simulink model "gm_uz_count_switching"  (R2024a)
settings: Solver=FixedStepDiscrete  StartTime=0.0  StopTime=350e-6  RelTol=1e-3
libraries: hdlsllib x9, simulink x1
settings Model: Creator=josef  LastModifiedBy=josef
settings SolverCC: AlgebraicLoopSolver=TrustRegion
settings DataIOCC: LimitDataPoints=on  SaveOutput=off  SaveTime=off
settings OptimizationCC: BlockReduction=off  ConditionallyExecuteInputs=off  DefaultParameterBehavior=Inlined  InheritOutputTypeSmallerThanSingle=on  LifeSpan=inf
settings DebuggingCC: AlgebraicLoopMsg=error  InheritedTsInSrcMsg=none  SingleTaskRateTransMsg=error  UnconnectedInputMsg=warning  UnconnectedOutputMsg=warning  UnconnectedLineMsg=warning  AllowSymbolicDim=off  StrictBusMsg=ErrorOnBusTreatedAsVector  SFUnexpectedBacktrackingDiag=warning  SFNoUnconditionalDefaultTransitionDiag=warning  SFExecutionAtInitializationDiag=none  ArithmeticOperatorsInVariantConditions=warning
settings HardwareCC: ProdBitPerPointer=32  ProdBitPerSizeT=32  ProdBitPerPtrDiffT=32  ProdLargestAtomicFloat=None  ProdIntDivRoundTo=Undefined  ProdEndianess=Unspecified  ProdWordSize=32  ProdHWDeviceType=ASIC/FPGA->ASIC/FPGA  ProdEqTarget=off
settings ModelReferenceCC: EnableRefExpFcnMdlSchedulingChecks=on
settings SFSimCC: SimUseLocalCustomCode=off  CustomCodeUndefinedFunction=UseInterfaceOnly
settings RTWCC: RTWUseLocalCustomCode=off  GPUComputeCapability=3.5
settings CodeAppCC: StateflowObjectComments=on
settings GRTTargetCC: TargetLangStandard=C89/C90 (ANSI)
settings ConfigComp: CovScope=ReferencedModels  CovMetricSettings=dw  CovSaveCumulativeToWorkspaceVar=on  CovSaveSingleToWorkspaceVar=on  CovExternalEMLEnable=off  CovSFcnEnable=off

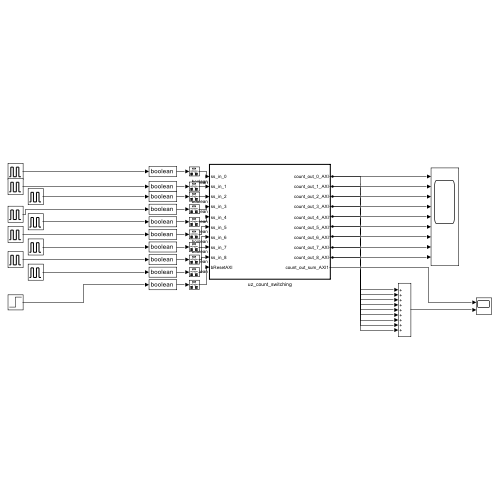
[thumbnail: Simulink's stored preview of the top-level diagram]
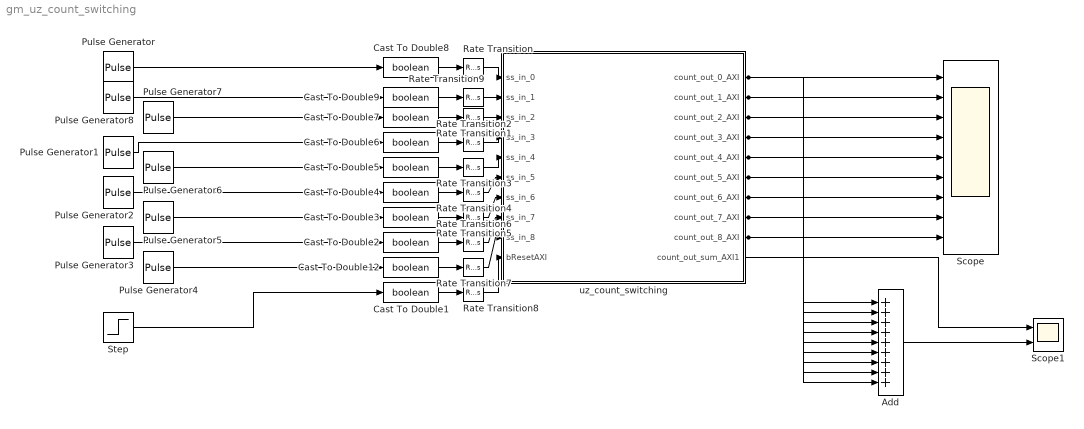
== system gm_uz_count_switching ==
  Add : Sum  Inputs=+++++++++
  Cast To Double{1..9,12} (10 alike) : DataTypeConversion  OutDataTypeStr=boolean  SaturateOnIntegerOverflow=off  RndMeth=Floor
  Pulse Generator{,1..5,7..8} (8 alike) : DiscretePulseGenerator  PulseType=Time based  Period=100e-6  PulseWidth=5
  Pulse Generator6 : DiscretePulseGenerator  PulseType=Time based  Period=50e-6  PulseWidth=5
  Rate Transition{,1..9} (10 alike) : RateTransition  OutPortSampleTime=1/100000000
  Scope : Scope  NumInputPorts=9
  Scope1 : Scope  NumInputPorts=2
  Step : Step  Time=2e-4  SampleTime=0
  uz_count_switching : Subsystem  TreatAsAtomicUnit=on
  wires:
  Pulse Generator8/1 -> Cast To Double9/1
  Cast To Double9/1 -> Rate Transition9/1
  Rate Transition9/1 -> uz_count_switching/2(ss_in_1)
  Rate Transition8/1 -> uz_count_switching/10(bResetAXI)
  Rate Transition7/1 -> uz_count_switching/9(ss_in_8)
  Rate Transition6/1 -> uz_count_switching/8(ss_in_7)
  Rate Transition5/1 -> uz_count_switching/7(ss_in_6)
  Rate Transition4/1 -> uz_count_switching/6(ss_in_5)
  Rate Transition3/1 -> uz_count_switching/5(ss_in_4)
  Rate Transition2/1 -> uz_count_switching/4(ss_in_3)
  Rate Transition1/1 -> uz_count_switching/3(ss_in_2)
  Cast To Double8/1 -> Rate Transition/1
  Cast To Double7/1 -> Rate Transition1/1
  Cast To Double6/1 -> Rate Transition2/1
  Cast To Double5/1 -> Rate Transition3/1
  Cast To Double4/1 -> Rate Transition4/1
  Cast To Double3/1 -> Rate Transition5/1
  Cast To Double2/1 -> Rate Transition6/1
  Cast To Double1/1 -> Rate Transition8/1
  Cast To Double12/1 -> Rate Transition7/1
  Rate Transition/1 -> uz_count_switching/1(ss_in_0)
  Pulse Generator5/1 -> Cast To Double3/1
  Pulse Generator6/1 -> Cast To Double5/1
  Pulse Generator7/1 -> Cast To Double7/1
  Pulse Generator4/1 -> Cast To Double12/1
  Pulse Generator3/1 -> Cast To Double2/1
  Pulse Generator2/1 -> Cast To Double4/1
  Pulse Generator1/1 -> Cast To Double6/1
  Pulse Generator/1 -> Cast To Double8/1
  Step/1 -> Cast To Double1/1
  Add/1 -> Scope1/2
  uz_count_switching/10(count_out_sum_AXI1) -> Scope1/1
  uz_count_switching/9(count_out_8_AXI) -> Scope/9, Add/9
  uz_count_switching/8(count_out_7_AXI) -> Scope/8, Add/8
  uz_count_switching/7(count_out_6_AXI) -> Scope/7, Add/7
  uz_count_switching/6(count_out_5_AXI) -> Scope/6, Add/6
  uz_count_switching/5(count_out_4_AXI) -> Scope/5, Add/5
  uz_count_switching/4(count_out_3_AXI) -> Scope/4, Add/4
  uz_count_switching/3(count_out_2_AXI) -> Scope/3, Add/3
  uz_count_switching/2(count_out_1_AXI) -> Scope/2, Add/2
  uz_count_switching/1(count_out_0_AXI) -> Scope/1, Add/1

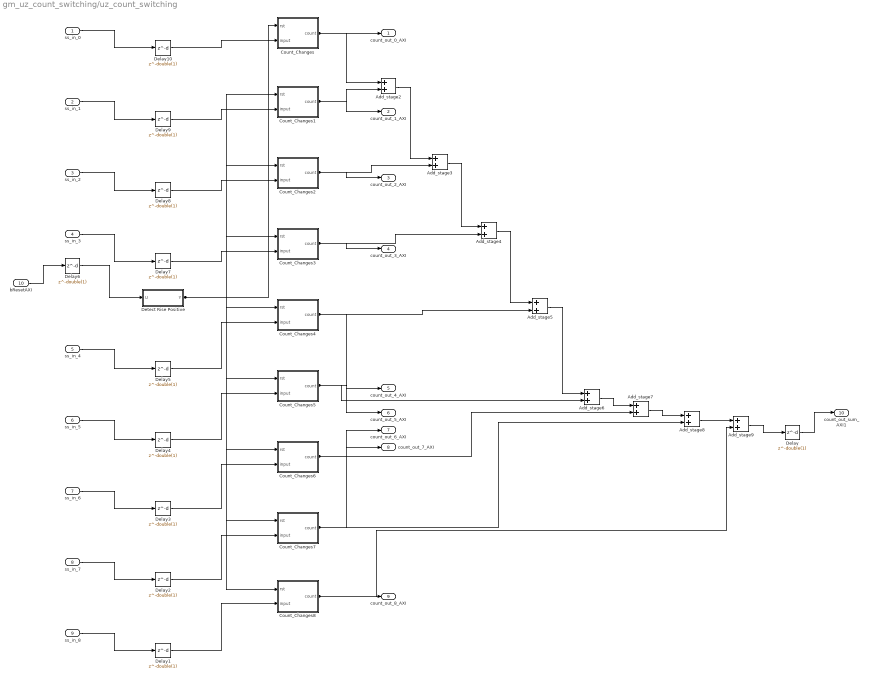
== system gm_uz_count_switching/uz_count_switching ==
  ss_in_0 : Inport  OutDataTypeStr=boolean  PortDimensions=1  SampleTime=1e-08
  ss_in_1 : Inport  Port=2  OutDataTypeStr=boolean  PortDimensions=1  SampleTime=1e-08
  ss_in_2 : Inport  Port=3  OutDataTypeStr=boolean  PortDimensions=1  SampleTime=1e-08
  ss_in_3 : Inport  Port=4  OutDataTypeStr=boolean  PortDimensions=1  SampleTime=1e-08
  ss_in_4 : Inport  Port=5  OutDataTypeStr=boolean  PortDimensions=1  SampleTime=1e-08
  ss_in_5 : Inport  Port=6  OutDataTypeStr=boolean  PortDimensions=1  SampleTime=1e-08
  ss_in_6 : Inport  Port=7  OutDataTypeStr=boolean  PortDimensions=1  SampleTime=1e-08
  ss_in_7 : Inport  Port=8  OutDataTypeStr=boolean  PortDimensions=1  SampleTime=1e-08
  ss_in_8 : Inport  Port=9  OutDataTypeStr=boolean  PortDimensions=1  SampleTime=1e-08
  bResetAXI : Inport  Port=10  OutDataTypeStr=boolean  PortDimensions=1  SampleTime=1e-08
  Add_stage2 : Sum  OutDataTypeStr=fixdt(0, 33, 0)  AccumDataTypeStr=uint32  SampleTime=1e-08
  Add_stage3 : Sum  OutDataTypeStr=fixdt(0, 34, 0)  AccumDataTypeStr=uint32  SampleTime=1e-08
  Add_stage4 : Sum  OutDataTypeStr=fixdt(0, 35, 0)  AccumDataTypeStr=uint32  SampleTime=1e-08
  Add_stage5 : Sum  OutDataTypeStr=fixdt(0, 36, 0)  AccumDataTypeStr=uint32  SampleTime=1e-08
  Add_stage6 : Sum  OutDataTypeStr=fixdt(0, 37, 0)  AccumDataTypeStr=uint32  SampleTime=1e-08
  Add_stage7 : Sum  OutDataTypeStr=fixdt(0, 38, 0)  AccumDataTypeStr=uint32  SampleTime=1e-08
  Add_stage8 : Sum  OutDataTypeStr=fixdt(0, 39, 0)  AccumDataTypeStr=uint32  SampleTime=1e-08
  Add_stage9 : Sum  OutDataTypeStr=uint32  AccumDataTypeStr=uint32  SampleTime=1e-08
  Count_Changes : Subsystem
  Count_Changes1 : Subsystem
  Count_Changes2 : Subsystem
  Count_Changes3 : Subsystem
  Count_Changes4 : Subsystem
  Count_Changes5 : Subsystem
  Count_Changes6 : Subsystem
  Count_Changes7 : Subsystem
  Count_Changes8 : Subsystem
  Delay{,1..10} (11 alike) : Delay  DelayLength=double(1)  InitialCondition=0  SampleTime=1e-08
  Detect Rise Positive : Subsystem  mask(Detect Rise Positive){vinit=double(0), InputProcessing=Elements as channels (sample based), OutDataTypeStr=boolean}
      mask prompts: vinit "Simulink:masks:InitialCondition_MP"; InputProcessing "Simulink:masks:InputProcessing_MP"; OutDataTypeStr "Simulink:masks:OutputDataType_MP"
      mask help: Simulink:masks:DetectRisePositive_MD
      mask init:
      | InputProcessing = 'Elements as channels (sample based)';
      | OutDataTypeStr = 'boolean';
      | vinit = double(0);
      mask TypeOptions InputProcessing: Simulink:masks:ColumnsAsChannelsFrameBased | Simulink:masks:ElementsAsChannelsSampleBased
      mask TypeOptions OutDataTypeStr: Simulink:masks:uint8 | Simulink:masks:boolean
      mask Display: fprintf('U > 0\n&  NOT\nU/z > 0')
  count_out_0_AXI : Outport  SampleTime=1e-08  VectorParamsAs1DForOutWhenUnconnected=off
  count_out_1_AXI : Outport  Port=2  SampleTime=1e-08  VectorParamsAs1DForOutWhenUnconnected=off
  count_out_2_AXI : Outport  Port=3  SampleTime=1e-08  VectorParamsAs1DForOutWhenUnconnected=off
  count_out_3_AXI : Outport  Port=4  SampleTime=1e-08  VectorParamsAs1DForOutWhenUnconnected=off
  count_out_4_AXI : Outport  Port=5  SampleTime=1e-08  VectorParamsAs1DForOutWhenUnconnected=off
  count_out_5_AXI : Outport  Port=6  SampleTime=1e-08  VectorParamsAs1DForOutWhenUnconnected=off
  count_out_6_AXI : Outport  Port=7  SampleTime=1e-08  VectorParamsAs1DForOutWhenUnconnected=off
  count_out_7_AXI : Outport  Port=8  SampleTime=1e-08  VectorParamsAs1DForOutWhenUnconnected=off
  count_out_8_AXI : Outport  Port=9  SampleTime=1e-08  VectorParamsAs1DForOutWhenUnconnected=off
  count_out_sum_AXI1 : Outport  Port=10  SampleTime=1e-08  VectorParamsAs1DForOutWhenUnconnected=off
  wires:
  ss_in_0/1 -> Delay10/1
  ss_in_1/1 -> Delay9/1
  ss_in_2/1 -> Delay8/1
  ss_in_3/1 -> Delay7/1
  ss_in_4/1 -> Delay5/1
  ss_in_5/1 -> Delay4/1
  ss_in_6/1 -> Delay3/1
  ss_in_7/1 -> Delay2/1
  ss_in_8/1 -> Delay1/1
  bResetAXI/1 -> Delay6/1
  Add_stage9/1 -> Delay/1
  Count_Changes/1(count) -> Add_stage2/1, count_out_0_AXI/1
  Count_Changes1/1(count) -> Add_stage2/2, count_out_1_AXI/1
  Count_Changes2/1(count) -> Add_stage3/2, count_out_2_AXI/1
  Count_Changes3/1(count) -> Add_stage4/2, count_out_3_AXI/1
  Count_Changes4/1(count) -> Add_stage5/2, count_out_4_AXI/1
  Count_Changes5/1(count) -> Add_stage6/2, count_out_5_AXI/1
  Count_Changes6/1(count) -> Add_stage7/2, count_out_6_AXI/1
  Count_Changes7/1(count) -> Add_stage8/2, count_out_7_AXI/1
  Count_Changes8/1(count) -> Add_stage9/2, count_out_8_AXI/1
  Delay/1 -> count_out_sum_AXI1/1
  Delay1/1 -> Count_Changes8/2(input)
  Delay10/1 -> Count_Changes/2(input)
  Delay2/1 -> Count_Changes7/2(input)
  Delay3/1 -> Count_Changes6/2(input)
  Delay4/1 -> Count_Changes5/2(input)
  Delay5/1 -> Count_Changes4/2(input)
  Delay6/1 -> Detect Rise Positive/1(U)
  Delay7/1 -> Count_Changes3/2(input)
  Delay8/1 -> Count_Changes2/2(input)
  Delay9/1 -> Count_Changes1/2(input)
  Detect Rise Positive/1(Y) -> Count_Changes/1(rst), Count_Changes1/1(rst), Count_Changes2/1(rst), Count_Changes3/1(rst), Count_Changes4/1(rst), Count_Changes5/1(rst), Count_Changes6/1(rst), Count_Changes7/1(rst), Count_Changes8/1(rst)
  Add_stage2/1 -> Add_stage3/1
  Add_stage3/1 -> Add_stage4/1
  Add_stage4/1 -> Add_stage5/1
  Add_stage5/1 -> Add_stage6/1
  Add_stage6/1 -> Add_stage7/1
  Add_stage7/1 -> Add_stage8/1
  Add_stage8/1 -> Add_stage9/1

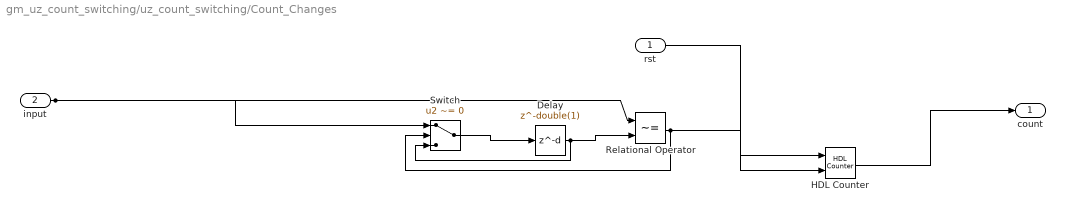
== system gm_uz_count_switching/uz_count_switching/Count_Changes ==
  rst : Inport  OutDataTypeStr=boolean  PortDimensions=1  SampleTime=1e-08
  input : Inport  Port=2  OutDataTypeStr=boolean  PortDimensions=1  SampleTime=1e-08
  Delay : Delay  DelayLength=double(1)  InitialCondition=0  SampleTime=1e-08
  HDL Counter : hdlsllib/Sources/HDL Counter  CountType=Free running  CountInit=0  CountStep=1  CountMax=25  CountFromType=Initial value  CountFrom=0  CountResetPort=on  CountLoadPort=off  CountEnbPort=on  CountDirPort=off  CountHitOutputPort=off  CountDataType=Unsigned  CountWordLen=CounterWordLength  CountFracLen=0  CountSampTime=1
  Relational Operator : RelationalOperator  Operator=~=  OutDataTypeStr=boolean  SampleTime=1e-08  InputSameDT=off
  Switch : Switch  Criteria=u2 ~= 0  Threshold=double(0)  OutDataTypeStr=boolean  SampleTime=1e-08  SaturateOnIntegerOverflow=off  InputSameDT=off
  count : Outport  SampleTime=1e-08
  wires:
  rst/1 -> HDL Counter/1
  input/1 -> Switch/1, Relational Operator/1
  Delay/1 -> Switch/3, Relational Operator/2
  HDL Counter/1 -> count/1
  Relational Operator/1 -> Switch/2, HDL Counter/2
  Switch/1 -> Delay/1

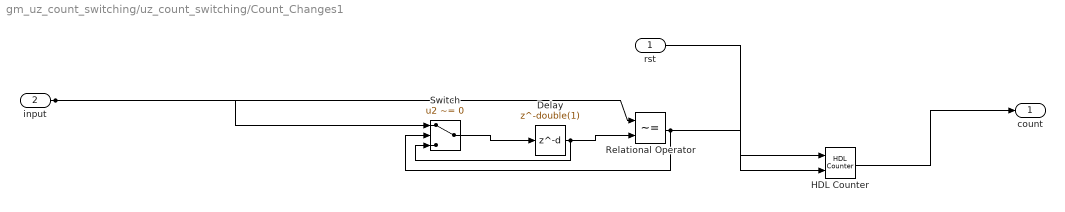
== system gm_uz_count_switching/uz_count_switching/Count_Changes1 ==
  rst : Inport  OutDataTypeStr=boolean  PortDimensions=1  SampleTime=1e-08
  input : Inport  Port=2  OutDataTypeStr=boolean  PortDimensions=1  SampleTime=1e-08
  Delay : Delay  DelayLength=double(1)  InitialCondition=0  SampleTime=1e-08
  HDL Counter : hdlsllib/Sources/HDL Counter  CountType=Free running  CountInit=0  CountStep=1  CountMax=25  CountFromType=Initial value  CountFrom=0  CountResetPort=on  CountLoadPort=off  CountEnbPort=on  CountDirPort=off  CountHitOutputPort=off  CountDataType=Unsigned  CountWordLen=CounterWordLength  CountFracLen=0  CountSampTime=1
  Relational Operator : RelationalOperator  Operator=~=  OutDataTypeStr=boolean  SampleTime=1e-08  InputSameDT=off
  Switch : Switch  Criteria=u2 ~= 0  Threshold=double(0)  OutDataTypeStr=boolean  SampleTime=1e-08  SaturateOnIntegerOverflow=off  InputSameDT=off
  count : Outport  SampleTime=1e-08
  wires:
  rst/1 -> HDL Counter/1
  input/1 -> Switch/1, Relational Operator/1
  Delay/1 -> Switch/3, Relational Operator/2
  HDL Counter/1 -> count/1
  Relational Operator/1 -> Switch/2, HDL Counter/2
  Switch/1 -> Delay/1

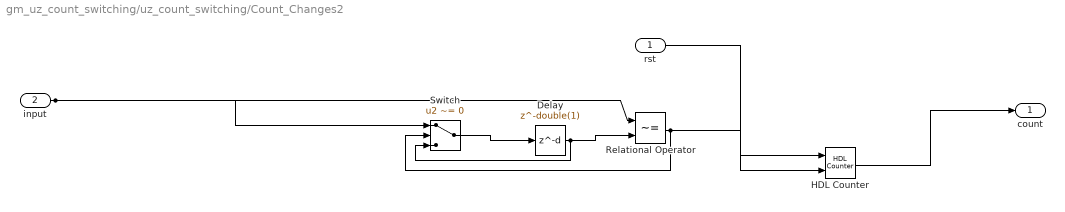
== system gm_uz_count_switching/uz_count_switching/Count_Changes2 ==
  rst : Inport  OutDataTypeStr=boolean  PortDimensions=1  SampleTime=1e-08
  input : Inport  Port=2  OutDataTypeStr=boolean  PortDimensions=1  SampleTime=1e-08
  Delay : Delay  DelayLength=double(1)  InitialCondition=0  SampleTime=1e-08
  HDL Counter : hdlsllib/Sources/HDL Counter  CountType=Free running  CountInit=0  CountStep=1  CountMax=25  CountFromType=Initial value  CountFrom=0  CountResetPort=on  CountLoadPort=off  CountEnbPort=on  CountDirPort=off  CountHitOutputPort=off  CountDataType=Unsigned  CountWordLen=CounterWordLength  CountFracLen=0  CountSampTime=1
  Relational Operator : RelationalOperator  Operator=~=  OutDataTypeStr=boolean  SampleTime=1e-08  InputSameDT=off
  Switch : Switch  Criteria=u2 ~= 0  Threshold=double(0)  OutDataTypeStr=boolean  SampleTime=1e-08  SaturateOnIntegerOverflow=off  InputSameDT=off
  count : Outport  SampleTime=1e-08
  wires:
  rst/1 -> HDL Counter/1
  input/1 -> Switch/1, Relational Operator/1
  Delay/1 -> Switch/3, Relational Operator/2
  HDL Counter/1 -> count/1
  Relational Operator/1 -> Switch/2, HDL Counter/2
  Switch/1 -> Delay/1

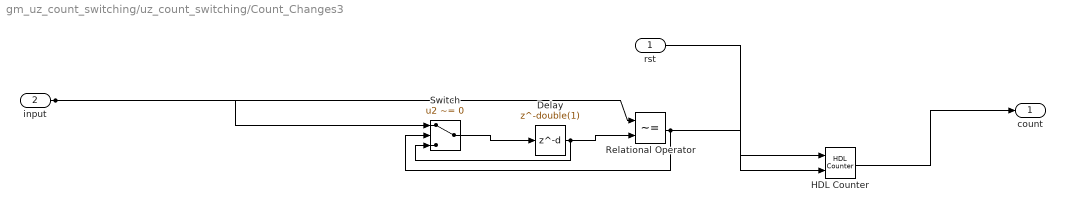
== system gm_uz_count_switching/uz_count_switching/Count_Changes3 ==
  rst : Inport  OutDataTypeStr=boolean  PortDimensions=1  SampleTime=1e-08
  input : Inport  Port=2  OutDataTypeStr=boolean  PortDimensions=1  SampleTime=1e-08
  Delay : Delay  DelayLength=double(1)  InitialCondition=0  SampleTime=1e-08
  HDL Counter : hdlsllib/Sources/HDL Counter  CountType=Free running  CountInit=0  CountStep=1  CountMax=25  CountFromType=Initial value  CountFrom=0  CountResetPort=on  CountLoadPort=off  CountEnbPort=on  CountDirPort=off  CountHitOutputPort=off  CountDataType=Unsigned  CountWordLen=CounterWordLength  CountFracLen=0  CountSampTime=1
  Relational Operator : RelationalOperator  Operator=~=  OutDataTypeStr=boolean  SampleTime=1e-08  InputSameDT=off
  Switch : Switch  Criteria=u2 ~= 0  Threshold=double(0)  OutDataTypeStr=boolean  SampleTime=1e-08  SaturateOnIntegerOverflow=off  InputSameDT=off
  count : Outport  SampleTime=1e-08
  wires:
  rst/1 -> HDL Counter/1
  input/1 -> Switch/1, Relational Operator/1
  Delay/1 -> Switch/3, Relational Operator/2
  HDL Counter/1 -> count/1
  Relational Operator/1 -> Switch/2, HDL Counter/2
  Switch/1 -> Delay/1

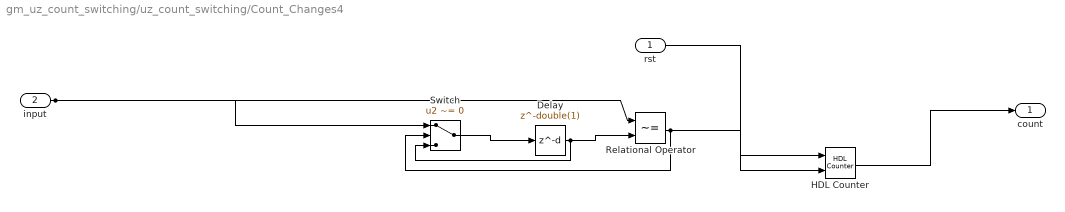
== system gm_uz_count_switching/uz_count_switching/Count_Changes4 ==
  rst : Inport  OutDataTypeStr=boolean  PortDimensions=1  SampleTime=1e-08
  input : Inport  Port=2  OutDataTypeStr=boolean  PortDimensions=1  SampleTime=1e-08
  Delay : Delay  DelayLength=double(1)  InitialCondition=0  SampleTime=1e-08
  HDL Counter : hdlsllib/Sources/HDL Counter  CountType=Free running  CountInit=0  CountStep=1  CountMax=25  CountFromType=Initial value  CountFrom=0  CountResetPort=on  CountLoadPort=off  CountEnbPort=on  CountDirPort=off  CountHitOutputPort=off  CountDataType=Unsigned  CountWordLen=CounterWordLength  CountFracLen=0  CountSampTime=1
  Relational Operator : RelationalOperator  Operator=~=  OutDataTypeStr=boolean  SampleTime=1e-08  InputSameDT=off
  Switch : Switch  Criteria=u2 ~= 0  Threshold=double(0)  OutDataTypeStr=boolean  SampleTime=1e-08  SaturateOnIntegerOverflow=off  InputSameDT=off
  count : Outport  SampleTime=1e-08
  wires:
  rst/1 -> HDL Counter/1
  input/1 -> Switch/1, Relational Operator/1
  Delay/1 -> Switch/3, Relational Operator/2
  HDL Counter/1 -> count/1
  Relational Operator/1 -> Switch/2, HDL Counter/2
  Switch/1 -> Delay/1

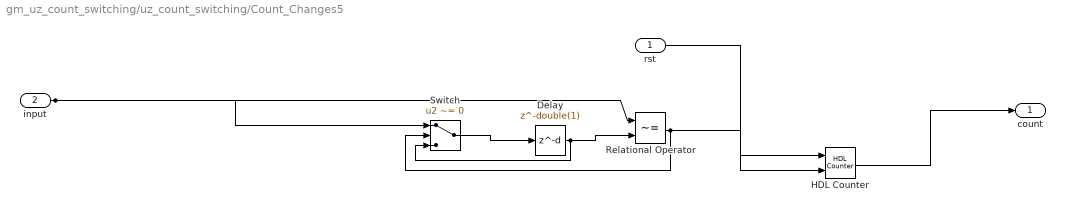
== system gm_uz_count_switching/uz_count_switching/Count_Changes5 ==
  rst : Inport  OutDataTypeStr=boolean  PortDimensions=1  SampleTime=1e-08
  input : Inport  Port=2  OutDataTypeStr=boolean  PortDimensions=1  SampleTime=1e-08
  Delay : Delay  DelayLength=double(1)  InitialCondition=0  SampleTime=1e-08
  HDL Counter : hdlsllib/Sources/HDL Counter  CountType=Free running  CountInit=0  CountStep=1  CountMax=25  CountFromType=Initial value  CountFrom=0  CountResetPort=on  CountLoadPort=off  CountEnbPort=on  CountDirPort=off  CountHitOutputPort=off  CountDataType=Unsigned  CountWordLen=CounterWordLength  CountFracLen=0  CountSampTime=1
  Relational Operator : RelationalOperator  Operator=~=  OutDataTypeStr=boolean  SampleTime=1e-08  InputSameDT=off
  Switch : Switch  Criteria=u2 ~= 0  Threshold=double(0)  OutDataTypeStr=boolean  SampleTime=1e-08  SaturateOnIntegerOverflow=off  InputSameDT=off
  count : Outport  SampleTime=1e-08
  wires:
  rst/1 -> HDL Counter/1
  input/1 -> Switch/1, Relational Operator/1
  Delay/1 -> Switch/3, Relational Operator/2
  HDL Counter/1 -> count/1
  Relational Operator/1 -> Switch/2, HDL Counter/2
  Switch/1 -> Delay/1

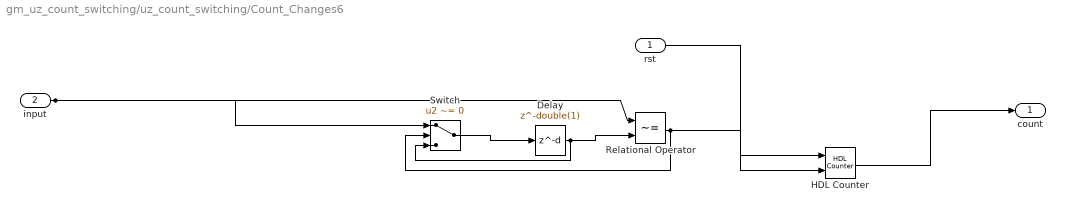
== system gm_uz_count_switching/uz_count_switching/Count_Changes6 ==
  rst : Inport  OutDataTypeStr=boolean  PortDimensions=1  SampleTime=1e-08
  input : Inport  Port=2  OutDataTypeStr=boolean  PortDimensions=1  SampleTime=1e-08
  Delay : Delay  DelayLength=double(1)  InitialCondition=0  SampleTime=1e-08
  HDL Counter : hdlsllib/Sources/HDL Counter  CountType=Free running  CountInit=0  CountStep=1  CountMax=25  CountFromType=Initial value  CountFrom=0  CountResetPort=on  CountLoadPort=off  CountEnbPort=on  CountDirPort=off  CountHitOutputPort=off  CountDataType=Unsigned  CountWordLen=CounterWordLength  CountFracLen=0  CountSampTime=1
  Relational Operator : RelationalOperator  Operator=~=  OutDataTypeStr=boolean  SampleTime=1e-08  InputSameDT=off
  Switch : Switch  Criteria=u2 ~= 0  Threshold=double(0)  OutDataTypeStr=boolean  SampleTime=1e-08  SaturateOnIntegerOverflow=off  InputSameDT=off
  count : Outport  SampleTime=1e-08
  wires:
  rst/1 -> HDL Counter/1
  input/1 -> Switch/1, Relational Operator/1
  Delay/1 -> Switch/3, Relational Operator/2
  HDL Counter/1 -> count/1
  Relational Operator/1 -> Switch/2, HDL Counter/2
  Switch/1 -> Delay/1

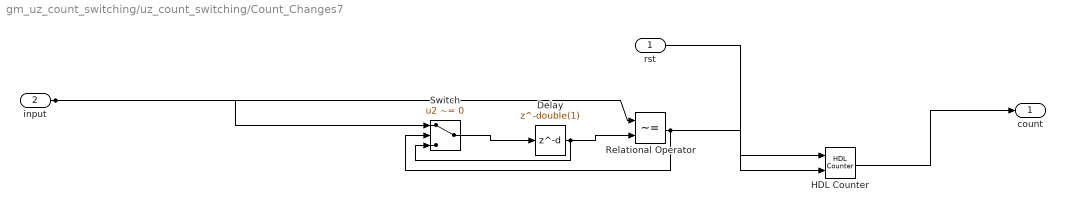
== system gm_uz_count_switching/uz_count_switching/Count_Changes7 ==
  rst : Inport  OutDataTypeStr=boolean  PortDimensions=1  SampleTime=1e-08
  input : Inport  Port=2  OutDataTypeStr=boolean  PortDimensions=1  SampleTime=1e-08
  Delay : Delay  DelayLength=double(1)  InitialCondition=0  SampleTime=1e-08
  HDL Counter : hdlsllib/Sources/HDL Counter  CountType=Free running  CountInit=0  CountStep=1  CountMax=25  CountFromType=Initial value  CountFrom=0  CountResetPort=on  CountLoadPort=off  CountEnbPort=on  CountDirPort=off  CountHitOutputPort=off  CountDataType=Unsigned  CountWordLen=CounterWordLength  CountFracLen=0  CountSampTime=1
  Relational Operator : RelationalOperator  Operator=~=  OutDataTypeStr=boolean  SampleTime=1e-08  InputSameDT=off
  Switch : Switch  Criteria=u2 ~= 0  Threshold=double(0)  OutDataTypeStr=boolean  SampleTime=1e-08  SaturateOnIntegerOverflow=off  InputSameDT=off
  count : Outport  SampleTime=1e-08
  wires:
  rst/1 -> HDL Counter/1
  input/1 -> Switch/1, Relational Operator/1
  Delay/1 -> Switch/3, Relational Operator/2
  HDL Counter/1 -> count/1
  Relational Operator/1 -> Switch/2, HDL Counter/2
  Switch/1 -> Delay/1

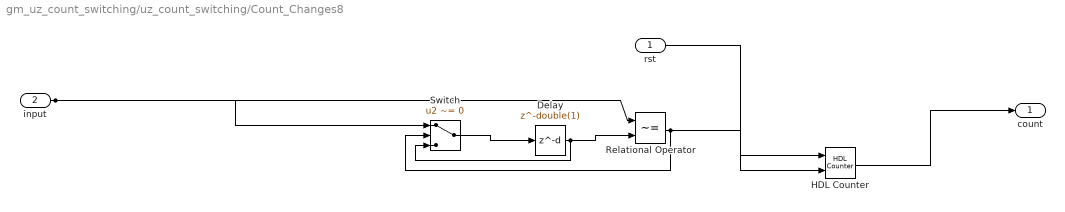
== system gm_uz_count_switching/uz_count_switching/Count_Changes8 ==
  rst : Inport  OutDataTypeStr=boolean  PortDimensions=1  SampleTime=1e-08
  input : Inport  Port=2  OutDataTypeStr=boolean  PortDimensions=1  SampleTime=1e-08
  Delay : Delay  DelayLength=double(1)  InitialCondition=0  SampleTime=1e-08
  HDL Counter : hdlsllib/Sources/HDL Counter  CountType=Free running  CountInit=0  CountStep=1  CountMax=25  CountFromType=Initial value  CountFrom=0  CountResetPort=on  CountLoadPort=off  CountEnbPort=on  CountDirPort=off  CountHitOutputPort=off  CountDataType=Unsigned  CountWordLen=CounterWordLength  CountFracLen=0  CountSampTime=1
  Relational Operator : RelationalOperator  Operator=~=  OutDataTypeStr=boolean  SampleTime=1e-08  InputSameDT=off
  Switch : Switch  Criteria=u2 ~= 0  Threshold=double(0)  OutDataTypeStr=boolean  SampleTime=1e-08  SaturateOnIntegerOverflow=off  InputSameDT=off
  count : Outport  SampleTime=1e-08
  wires:
  rst/1 -> HDL Counter/1
  input/1 -> Switch/1, Relational Operator/1
  Delay/1 -> Switch/3, Relational Operator/2
  HDL Counter/1 -> count/1
  Relational Operator/1 -> Switch/2, HDL Counter/2
  Switch/1 -> Delay/1

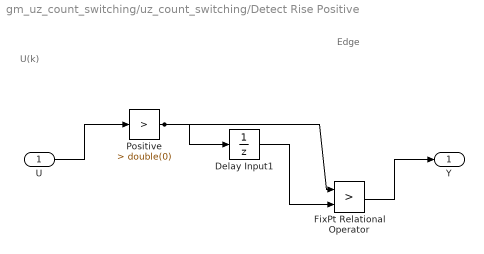
== system gm_uz_count_switching/uz_count_switching/Detect Rise Positive ==
  note: U(k)
  note: Edge
  U : Inport  OutDataTypeStr=boolean  SampleTime=1e-08
  Delay Input1 : UnitDelay  SampleTime=1e-08
  FixPt Relational Operator : RelationalOperator  Operator=>  OutDataTypeStr=boolean  SampleTime=1e-08  InputSameDT=off
  Positive : simulink/Logic and Bit Operations/Compare To Constant  relop=>  const=double(0)  OutDataTypeStr=boolean
  Y : Outport  SampleTime=1e-08
  wires:
  U/1 -> Positive/1
  Delay Input1/1 -> FixPt Relational Operator/2
  FixPt Relational Operator/1 -> Y/1
  Positive/1 -> FixPt Relational Operator/1, Delay Input1/1
